simulink model "sys"  (R2017a)
settings: Solver=VariableStepAuto  StartTime=0.0  StopTime=10.0  RelTol=1e-3
values from neighbouring files (symbols this model uses):
  Dp = 5.52e-03    (= 0.00552)    [FurutaSymb3.m]
  Dr = 6.0e-03    (= 0.006)    [FurutaSymb3.m]
  g = 9.81    [FurutaSymb3.m]    (also in Linear.m)
  Jp = 0.01    [FurutaSymb3.m]
  Jr = 0.05    [FurutaSymb3.m]
  Jt = Jp*mp*Lr*Lr+Jr*Jp + 0.25 *Jr*mp*Lp*Lp    (= 0.000561822931286)    [FurutaSymb3.m]
  km = 0.01    [FurutaSymb3.m]
  Lp = 239.73e-3    (= 0.23973)    [FurutaSymb3.m]
  Lr = 230.45e-3    (= 0.23045)    [FurutaSymb3.m]
  mp = 0.04948    [FurutaSymb3.m]    (also in Linear.m)
  Rm = 12.38    [FurutaSymb3.m]
  X0 = pi    (= 3.14159265359)    [FurutaSymb3.m]
settings Model: Creator=felip  LastModifiedBy=felip

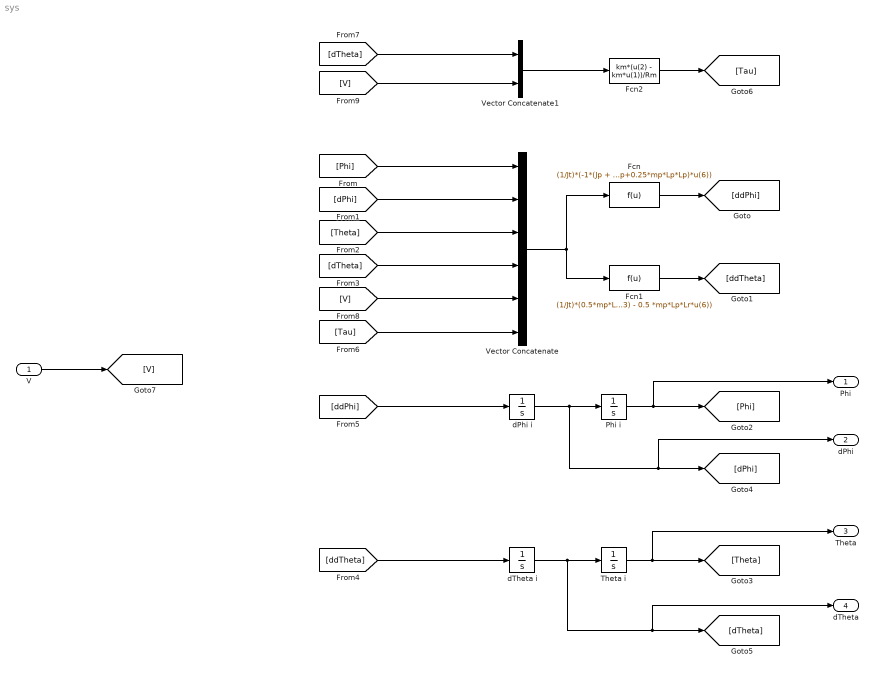
== system sys ==
  "V " : Inport
  Fcn : Fcn  Expr=(1/Jt)*(-1*(Jp + 0.25*mp*Lp*Lp)*Dr*u(2) + 0.5*mp*Lp*Lr*Dp*u(4) + 0.25 *mp*mp*Lp*Lp*g*u(3) + (Jp+0.25*mp*Lp*Lp)*u(6))
  Fcn1 : Fcn  Expr=(1/Jt)*(0.5*mp*Lp*Lr*Dr*u(2) - (Jr + mp*Lr*Lr)*Dp*u(4) - 0.5*mp*Lp*g*(Jr+mp*Lr*Lr)*u(3) - 0.5 *mp*Lp*Lr*u(6))
  Fcn2 : Fcn  Expr=km*(u(2) - km*u(1))/Rm
  Phi i : Integrator
  Theta i : Integrator  InitialCondition=X0
  Vector Concatenate : Concatenate  NumInputs=6
  Vector Concatenate1 : Concatenate
  dPhi i : Integrator
  dTheta i : Integrator
  Phi : Outport
  dPhi : Outport  Port=2
  Theta : Outport  Port=3
  dTheta : Outport  Port=4
  wires:
  [ddTheta] -> dTheta i/1
  Theta i/1 -> Theta/1, [Theta]
  [Phi] -> Vector Concatenate/1
  [ddPhi] -> dPhi i/1
  [dTheta] -> Vector Concatenate/4
  [V] -> Vector Concatenate/5
  Phi i/1 -> Phi/1, [Phi]
  dTheta i/1 -> dTheta/1, [dTheta], Theta i/1
  dPhi i/1 -> dPhi/1, [dPhi], Phi i/1
  [Theta] -> Vector Concatenate/3
  [dPhi] -> Vector Concatenate/2
  [dTheta] -> Vector Concatenate1/1
  Fcn1/1 -> [ddTheta]
  [V] -> Vector Concatenate1/2
  "V "/1 -> [V]
  Vector Concatenate/1 -> Fcn/1, Fcn1/1
  [Tau] -> Vector Concatenate/6
  Vector Concatenate1/1 -> Fcn2/1
  Fcn2/1 -> [Tau]
  Fcn/1 -> [ddPhi]
